simulink library "phase_shift_filter"  (R2025b)
settings: Solver=VariableStepAuto  StartTime=0.0  StopTime=10.0  RelTol=1e-3
undefined symbols (not defined in the file): freq, ts
settings Model: Creator=dbagn  LastModifiedBy=dbagn

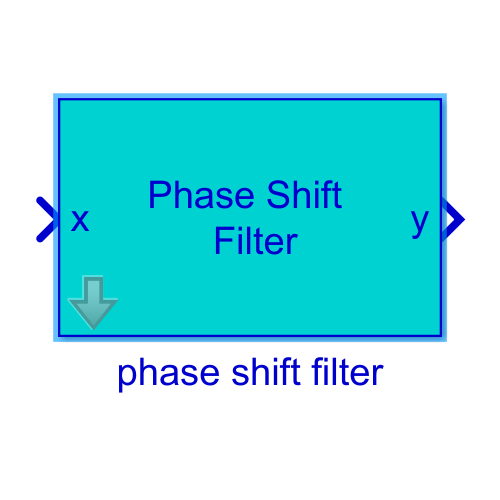
[thumbnail: Simulink's stored preview of the top-level diagram]
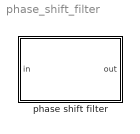
== system phase_shift_filter ==
  phase shift filter : Subsystem  mask{f=freq, ts=ts}
      mask prompts: f "frequency at 90 deg shift"; ts "sampling time"
      mask Display:
      | disp('Phase Shift \n Filter');
      | port_label('input', 1, 'x');
      | port_label('output', 1, 'y');

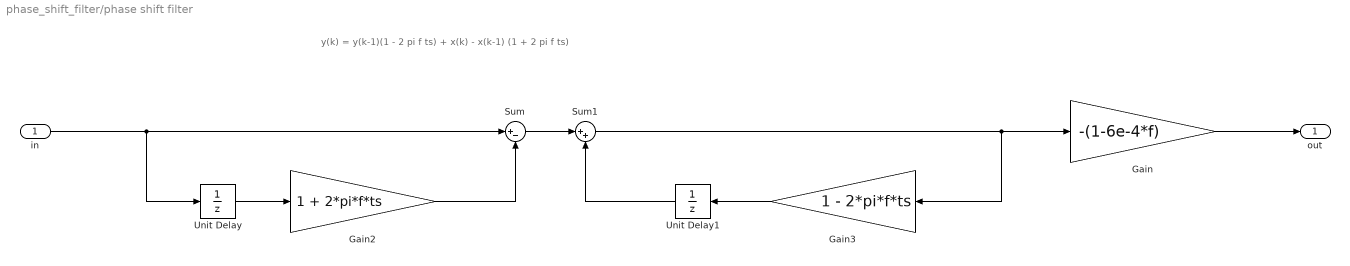
== system phase_shift_filter/phase shift filter ==
  note: y(k) = y(k-1)(1 - 2 pi f ts) + x(k) - x(k-1) (1 + 2 pi f ts)
  in : Inport
  Gain : Gain  Gain=-(1-6e-4*f)
  Gain2 : Gain  Gain=1 + 2*pi*f*ts
  Gain3 : Gain  Gain=1 - 2*pi*f*ts
  Sum : Sum  Inputs=|+-
  Sum1 : Sum  Inputs=|++
  Unit Delay : UnitDelay  SampleTime=-1  HasFrameUpgradeWarning=on
  Unit Delay1 : UnitDelay  SampleTime=-1  HasFrameUpgradeWarning=on
  out : Outport
  wires:
  Unit Delay/1 -> Gain2/1
  Sum/1 -> Sum1/1
  Unit Delay1/1 -> Sum1/2
  in/1 -> Sum/1, Unit Delay/1
  Gain2/1 -> Sum/2
  Gain3/1 -> Unit Delay1/1
  Sum1/1 -> Gain3/1, Gain/1
  Gain/1 -> out/1
